simulink model "Lyapanov"  (R2021a)
settings: Solver=VariableStepAuto  StartTime=0.0  StopTime=1000  RelTol=1e-3
values from neighbouring files (symbols this model uses):
  a0 = 1/(tau1*tau2)    (= 1.4940706006e-05)    [TA1.m]
  a1 = (tau1+tau2+A*R2)/(tau1*tau2)    (= 0.0166321059812)    [TA1.m]
  b = R2/(tau1*tau2)    (= 1.64347766066e-05)    [TA1.m]
  gamma = 3000    [TA1.m]
settings Model: Creator=ASUS  LastModifiedBy=ASUS

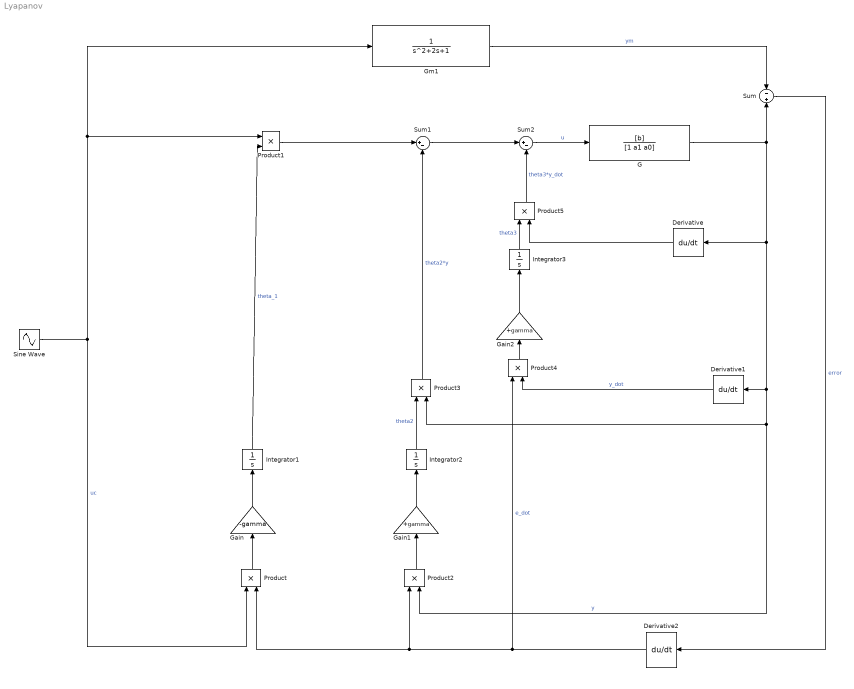
== system Lyapanov ==
  Derivative : Derivative
  Derivative1 : Derivative
  Derivative2 : Derivative
  G : TransferFcn  Numerator=[b]  Denominator=[1 a1 a0]
  Gain : Gain  Gain=-gamma
  Gain1 : Gain  Gain=+gamma
  Gain2 : Gain  Gain=+gamma
  Gm1 : TransferFcn
  Integrator1 : Integrator
  Integrator2 : Integrator
  Integrator3 : Integrator
  Product{,1..5} (6 alike) : Product
  Sine Wave : Sin  Frequency=0.1  SampleTime=0
  Sum : Sum  Inputs=-+
  Sum1 : Sum  Inputs=|+-
  Sum2 : Sum  Inputs=|+-
  wires:
  Product3/1 -> Sum1/2  "theta2*y"
  G/1 -> Sum/2, Derivative1/1, Product2/2, Product3/2, Derivative/1  "y"
  Integrator2/1 -> Product3/1  "theta2"
  Gain/1 -> Integrator1/1
  Integrator1/1 -> Product1/2  "theta_1"
  Gain1/1 -> Integrator2/1
  Product/1 -> Gain/1
  Gm1/1 -> Sum/1  "ym"
  Derivative/1 -> Product5/2
  Sum2/1 -> G/1  "u"
  Product1/1 -> Sum1/1
  Product5/1 -> Sum2/2  "theta3*y_dot"
  Product4/1 -> Gain2/1
  Sine Wave/1 -> Product/1, Gm1/1, Product1/1  "uc"
  Integrator3/1 -> Product5/1  "theta3"
  Sum1/1 -> Sum2/1
  Gain2/1 -> Integrator3/1
  Sum/1 -> Derivative2/1  "error"
  Derivative1/1 -> Product4/2  "y_dot"
  Product2/1 -> Gain1/1
  Derivative2/1 -> Product4/1, Product2/1, Product/2  "e_dot"
